simulink model "simAIDC"  (R2023b)
settings: Solver=VariableStepAuto  StartTime=0.0  StopTime=100.0  RelTol=1e-3
undefined symbols (not defined in the file or in its folder): beta, D_d, dragcoeff, G_d, gamma, K_D, K_P, Lambda, M_d, pos_init, pp, quat_init, snake, theta_init, x_init
libraries: dspindex x2
settings Model: Creator=sarava  LastModifiedBy=asker
settings SolverCC: AlgebraicLoopSolver=TrustRegion
settings DataIOCC: ReturnWorkspaceOutputs=off
settings DebuggingCC: UnconnectedInputMsg=warning  UnconnectedOutputMsg=warning  UnconnectedLineMsg=warning  ArithmeticOperatorsInVariantConditions=warning
settings ModelReferenceCC: EnableRefExpFcnMdlSchedulingChecks=on
settings SFSimCC: SimUseLocalCustomCode=off  CustomCodeUndefinedFunction=UseInterfaceOnly
settings RTWCC: RTWUseLocalCustomCode=off

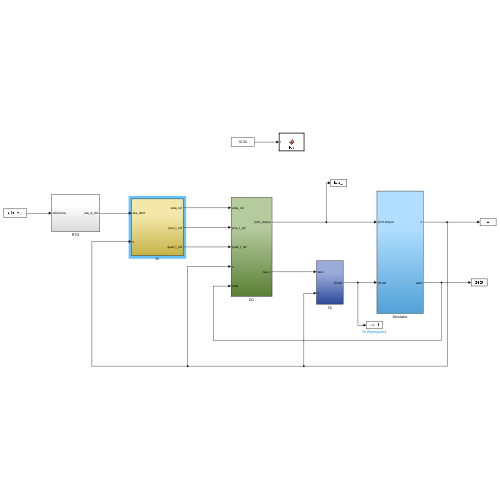
[thumbnail: Simulink's stored preview of the top-level diagram]
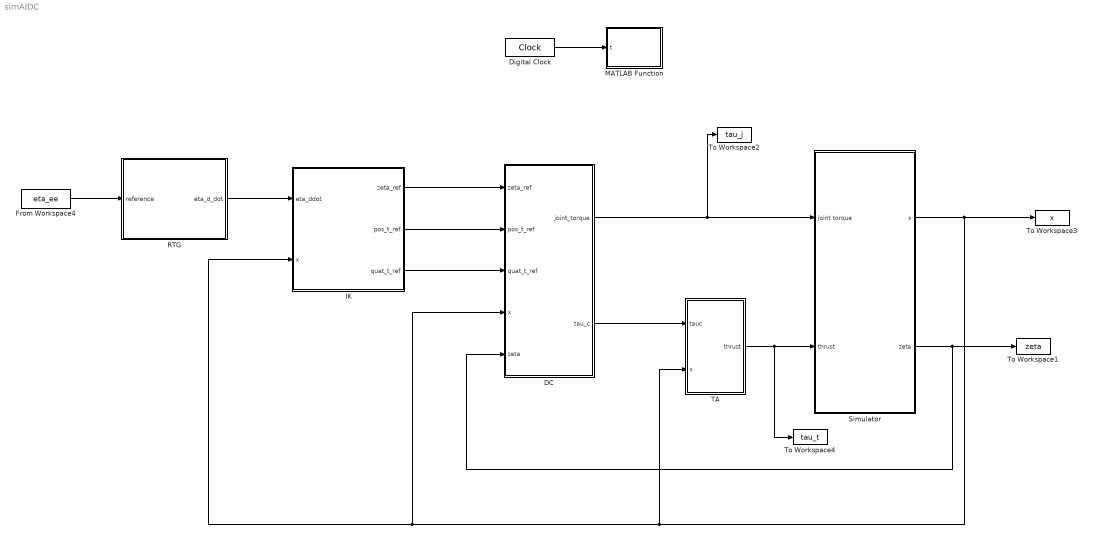
== system simAIDC ==
  DC : Subsystem
  Digital Clock : DigitalClock
  From Workspace4 : FromWorkspace  VariableName=eta_ee
  IK : Subsystem
  MATLAB Function : MATLAB Function  TreatAsAtomicUnit=on
  RTG : Subsystem
  Simulator : Subsystem
  TA : Subsystem
  To Workspace1 : ToWorkspace  VariableName=zeta  SaveFormat=Timeseries  SampleTime=-1
  To Workspace2 : ToWorkspace  VariableName=tau_j  SaveFormat=Timeseries  SampleTime=-1
  To Workspace3 : ToWorkspace  VariableName=x  SaveFormat=Timeseries  SampleTime=-1
  To Workspace4 : ToWorkspace  VariableName=tau_t  SaveFormat=Timeseries  SampleTime=-1
  wires:
  DC/2(tau_c) -> TA/1("tauc ")
  Digital Clock/1 -> MATLAB Function/1(t)
  Simulator/2(zeta) -> DC/5("zeta "), To Workspace1/1
  Simulator/1(x) -> IK/2(x), DC/4(x), TA/2("x "), To Workspace3/1
  IK/2(pos_t_ref) -> DC/2(pos_t_ref)
  IK/1(zeta_ref) -> DC/1(zeta_ref)
  IK/3(quat_t_ref) -> DC/3(quat_t_ref)
  From Workspace4/1 -> RTG/1(reference)
  RTG/1(eta_d_dot) -> IK/1(eta_ddot)
  DC/1(joint_torque) -> To Workspace2/1, Simulator/1(joint torque)
  TA/1(thrust) -> Simulator/2(thrust), To Workspace4/1

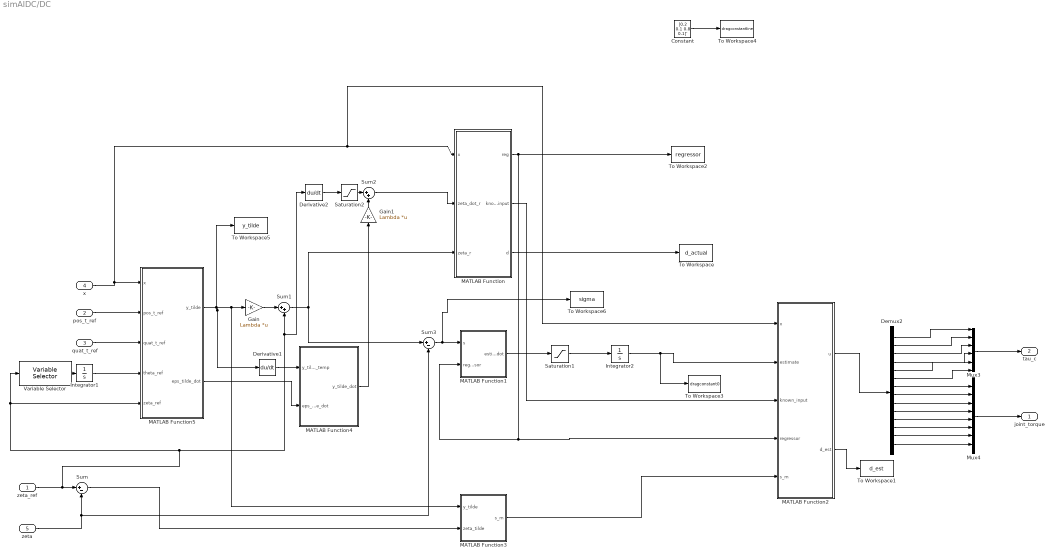
== system simAIDC/DC ==
  zeta_ref : Inport
  pos_t_ref : Inport  Port=2
  quat_t_ref : Inport  Port=3
  x : Inport  Port=4
  "zeta " : Inport  Port=5
  Constant : Constant  Value=[0.2 0.1 0.8 0.1]'
  Demux2 : Demux  Outputs=14
  Derivative1 : Derivative  CoefficientInTFapproximation=10
  Derivative2 : Derivative  CoefficientInTFapproximation=10
  Gain : Gain  Gain=Lambda  Multiplication=Matrix(K*u) (u vector)
  Gain1 : Gain  Gain=Lambda  Multiplication=Matrix(K*u) (u vector)
  Integrator1 : Integrator  InitialCondition=theta_init
  Integrator2 : Integrator  InitialCondition=[0 0 0 0]'
  MATLAB Function : MATLAB Function  TreatAsAtomicUnit=on
  MATLAB Function1 : MATLAB Function  TreatAsAtomicUnit=on
  MATLAB Function2 : MATLAB Function  TreatAsAtomicUnit=on
  MATLAB Function3 : MATLAB Function  TreatAsAtomicUnit=on
  MATLAB Function4 : MATLAB Function  TreatAsAtomicUnit=on
  MATLAB Function5 : MATLAB Function  TreatAsAtomicUnit=on
  Mux3 : Mux  Inputs=6
  Mux4 : Mux  Inputs=8
  Saturation1 : Saturate  UpperLimit=50  LowerLimit=-50  ZeroCross=off
  Saturation2 : Saturate  UpperLimit=20  LowerLimit=-20  ZeroCross=off
  Sum : Sum  Inputs=|+-
  Sum1 : Sum  Inputs=|++
  Sum2 : Sum  Inputs=|++
  Sum3 : Sum  Inputs=|+-
  To Workspace : ToWorkspace  VariableName=d_actual  SaveFormat=Timeseries  SampleTime=-1
  To Workspace1 : ToWorkspace  VariableName=d_est  SaveFormat=Timeseries  SampleTime=-1
  To Workspace2 : ToWorkspace  VariableName=regressor  SaveFormat=Timeseries  SampleTime=-1
  To Workspace3 : ToWorkspace  VariableName=dragconstant0  SaveFormat=Timeseries  SampleTime=-1
  To Workspace4 : ToWorkspace  VariableName=dragconstantline  SaveFormat=Timeseries  SampleTime=-1
  To Workspace5 : ToWorkspace  VariableName=y_tilde  SaveFormat=Timeseries  SampleTime=-1
  To Workspace6 : ToWorkspace  VariableName=sigma  SaveFormat=Timeseries  SampleTime=-1
  Variable Selector : dspindex/Variable Selector  NumInputs=1  rowsOrCols=Rows  IdxMode=Fixed  Elements=7:14  ZerOneIdxMode=One-based  errmode=Clip Index  FillMode=on  FillValues=0
  joint_torque : Outport  VectorParamsAs1DForOutWhenUnconnected=off
  tau_c : Outport  Port=2  VectorParamsAs1DForOutWhenUnconnected=off
  wires:
  x/1 -> MATLAB Function/1(x), MATLAB Function2/1(x), MATLAB Function5/1(x)
  pos_t_ref/1 -> MATLAB Function5/2(pos_t_ref)
  quat_t_ref/1 -> MATLAB Function5/3(quat_t_ref)
  zeta_ref/1 -> Derivative2/1, Sum1/2, Variable Selector/1, MATLAB Function5/5(zeta_ref), Sum/1
  "zeta "/1 -> Sum3/2, Sum/2
  Integrator1/1 -> MATLAB Function5/4(theta_ref)
  MATLAB Function5/1(y_tilde) -> MATLAB Function3/1(y_tilde), Gain/1, Derivative1/1, To Workspace5/1
  Gain/1 -> Sum1/1
  Sum1/1 -> Sum3/1, MATLAB Function/3(zeta_r)
  Saturation1/1 -> Integrator2/1
  MATLAB Function1/1(estimate_dot) -> Saturation1/1
  MATLAB Function3/1(s_m) -> MATLAB Function2/5(s_m)
  MATLAB Function2/1(u) -> Demux2/1
  Demux2/14 -> Mux4/8
  Demux2/4 -> Mux3/4
  Demux2/5 -> Mux3/5
  Demux2/12 -> Mux4/6
  Demux2/2 -> Mux3/2
  Demux2/9 -> Mux4/3
  Demux2/3 -> Mux3/3
  Demux2/13 -> Mux4/7
  Demux2/8 -> Mux4/2
  Demux2/6 -> Mux3/6
  Demux2/10 -> Mux4/4
  Demux2/7 -> Mux4/1
  Demux2/11 -> Mux4/5
  Demux2/1 -> Mux3/1
  Mux4/1 -> joint_torque/1
  Mux3/1 -> tau_c/1
  Variable Selector/1 -> Integrator1/1
  Integrator2/1 -> To Workspace3/1, MATLAB Function2/2(estimate)
  MATLAB Function/2(known_input) -> MATLAB Function2/3(known_input)
  MATLAB Function/1(reg) -> MATLAB Function1/2(regressor), MATLAB Function2/4(regressor), To Workspace2/1
  MATLAB Function5/2(eps_tilde_dot) -> MATLAB Function4/2(eps_tilde_dot)
  Derivative1/1 -> MATLAB Function4/1(y_tilde_dot_temp)
  MATLAB Function4/1(y_tilde_dot) -> Gain1/1
  Derivative2/1 -> Saturation2/1
  Saturation2/1 -> Sum2/1
  Gain1/1 -> Sum2/2
  Sum3/1 -> To Workspace6/1, MATLAB Function1/1(s)
  Sum2/1 -> MATLAB Function/2(zeta_dot_r)
  Sum/1 -> MATLAB Function3/2(zeta_tilde)
  MATLAB Function/3(d) -> To Workspace/1
  MATLAB Function2/2(d_est) -> To Workspace1/1
  Constant/1 -> To Workspace4/1

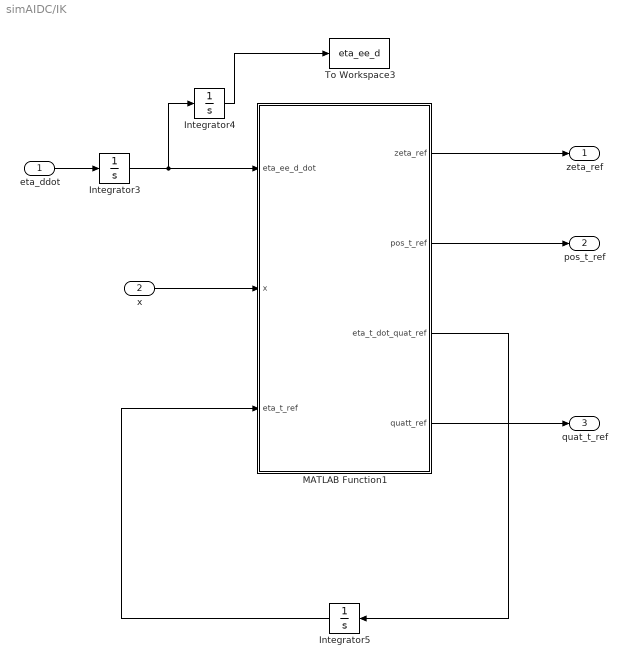
== system simAIDC/IK ==
  eta_ddot : Inport
  x : Inport  Port=2
  Integrator3 : Integrator
  Integrator4 : Integrator
  Integrator5 : Integrator  InitialCondition=[pos_init quat_init]'
  MATLAB Function1 : MATLAB Function  TreatAsAtomicUnit=on
  To Workspace3 : ToWorkspace  VariableName=eta_ee_d  SaveFormat=Timeseries  SampleTime=-1
  zeta_ref : Outport  VectorParamsAs1DForOutWhenUnconnected=off
  pos_t_ref : Outport  Port=2  VectorParamsAs1DForOutWhenUnconnected=off
  quat_t_ref : Outport  Port=3  VectorParamsAs1DForOutWhenUnconnected=off
  wires:
  MATLAB Function1/1(zeta_ref) -> zeta_ref/1
  x/1 -> MATLAB Function1/2(x)
  MATLAB Function1/2(pos_t_ref) -> pos_t_ref/1
  MATLAB Function1/3(eta_t_dot_quat_ref) -> Integrator5/1
  Integrator4/1 -> To Workspace3/1
  Integrator5/1 -> MATLAB Function1/3(eta_t_ref)
  MATLAB Function1/4(quatt_ref) -> quat_t_ref/1
  eta_ddot/1 -> Integrator3/1
  Integrator3/1 -> Integrator4/1, MATLAB Function1/1(eta_ee_d_dot)

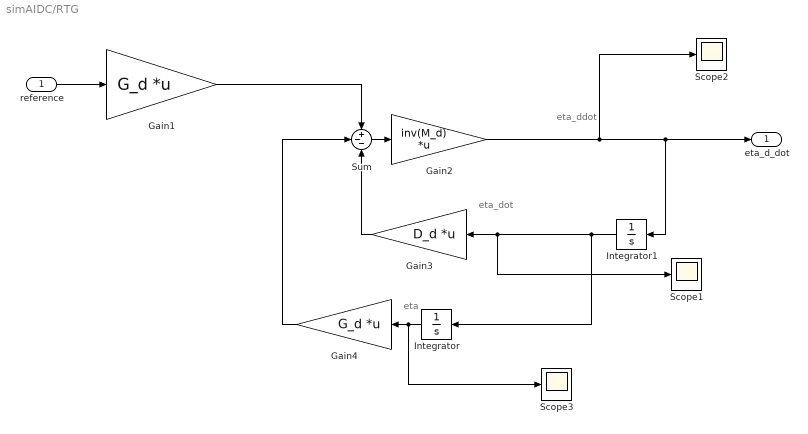
== system simAIDC/RTG ==
  note: eta_dot
  note: eta
  note: eta_ddot
  reference : Inport
  Gain1 : Gain  Gain=G_d  Multiplication=Matrix(K*u) (u vector)
  Gain2 : Gain  Gain=inv(M_d)  Multiplication=Matrix(K*u) (u vector)
  Gain3 : Gain  Gain=D_d  Multiplication=Matrix(K*u) (u vector)
  Gain4 : Gain  Gain=G_d  Multiplication=Matrix(K*u) (u vector)
  Integrator : Integrator
  Integrator1 : Integrator
  Scope1 : Scope
  Scope2 : Scope
  Scope3 : Scope
  Sum : Sum  Inputs=+--
  eta_d_dot : Outport  VectorParamsAs1DForOutWhenUnconnected=off
  wires:
  Gain2/1 -> Scope2/1, eta_d_dot/1, Integrator1/1
  Gain1/1 -> Sum/1
  Sum/1 -> Gain2/1
  reference/1 -> Gain1/1
  Integrator1/1 -> Integrator/1, Scope1/1, Gain3/1
  Integrator/1 -> Scope3/1, Gain4/1
  Gain3/1 -> Sum/3
  Gain4/1 -> Sum/2

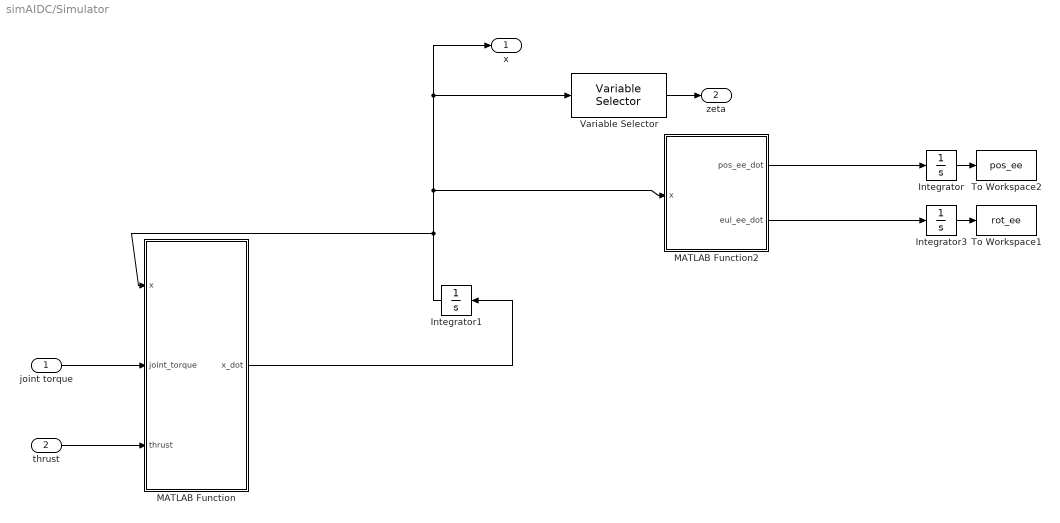
== system simAIDC/Simulator ==
  joint torque : Inport
  thrust : Inport  Port=2
  Integrator : Integrator
  Integrator1 : Integrator  InitialCondition=x_init
  Integrator3 : Integrator
  MATLAB Function : MATLAB Function  TreatAsAtomicUnit=on
  MATLAB Function2 : MATLAB Function  TreatAsAtomicUnit=on
  To Workspace1 : ToWorkspace  VariableName=rot_ee  SaveFormat=Timeseries  SampleTime=-1
  To Workspace2 : ToWorkspace  VariableName=pos_ee  SaveFormat=Timeseries  SampleTime=-1
  Variable Selector : dspindex/Variable Selector  NumInputs=1  rowsOrCols=Rows  IdxMode=Fixed  Elements=16:29  ZerOneIdxMode=One-based  errmode=Clip Index  FillMode=on  FillValues=0
  x : Outport  VectorParamsAs1DForOutWhenUnconnected=off
  zeta : Outport  Port=2  VectorParamsAs1DForOutWhenUnconnected=off
  wires:
  joint torque/1 -> MATLAB Function/2(joint_torque)
  thrust/1 -> MATLAB Function/3(thrust)
  Variable Selector/1 -> zeta/1
  MATLAB Function/1(x_dot) -> Integrator1/1
  Integrator1/1 -> Variable Selector/1, x/1, MATLAB Function2/1(x), MATLAB Function/1(x)
  Integrator/1 -> To Workspace2/1
  MATLAB Function2/1(pos_ee_dot) -> Integrator/1
  MATLAB Function2/2(eul_ee_dot) -> Integrator3/1
  Integrator3/1 -> To Workspace1/1

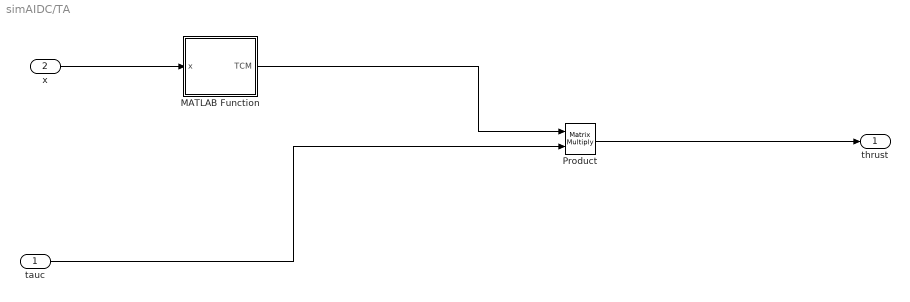
== system simAIDC/TA ==
  "tauc " : Inport
  "x " : Inport  Port=2
  MATLAB Function : MATLAB Function  TreatAsAtomicUnit=on
  Product : Product  Multiplication=Matrix(*)
  thrust : Outport  VectorParamsAs1DForOutWhenUnconnected=off
  wires:
  "x "/1 -> MATLAB Function/1(x)
  MATLAB Function/1(TCM) -> Product/1
  "tauc "/1 -> Product/2
  Product/1 -> thrust/1

== matlab function simAIDC/DC/MATLAB Function ==
  data: x input; zeta_dot_r input; reg output; known_input output; snake parameter; pp parameter; gamma parameter; beta parameter; zeta_r input; d output
function [reg, known_input,d] = regressor(x,zeta_dot_r,snake,pp, gamma, beta, zeta_r)

quat      =  x(4:7);
theta     =  x(8 : 6+snake.n);
zeta      =  x(7+snake.n : 11+2*snake.n);
[R, J]    =  comp_rot_jac(quat,theta,snake);
[c,d,g,D] = comp_cdg_adaptiv(J,R,theta,snake,pp,beta,gamma,zeta,zeta_r);
M = comp_mass(J,snake);




drag_matrix=zeros(14,4);
for i=1:snake.n
 drag_matrix=drag_matrix+J(:,:,i)'*D(:,:,i);
end



known_input= M*zeta_dot_r+c+g;

reg=drag_matrix;


end

== matlab function simAIDC/DC/MATLAB Function1 ==
  data: s input; regressor input; estimate_dot output; K_theta parameter
function estimate_dot = calc_estdot(s,regressor,K_theta)


estimate_dot=inv(K_theta)*regressor'*s;

end

== matlab function simAIDC/DC/MATLAB Function2 ==
  data: x input; estimate input; known_input input; regressor input; u output; s_m input; K_D parameter; snake parameter; d_est output
function [u,d_est]= input(x,estimate,known_input,regressor,s_m, K_D,snake)

quat      =  x(4:7);
theta     =  x(8 : 6+snake.n);

[~, J]    =  comp_rot_jac(quat,theta,snake);


B=comp_TCM(J,snake);
B_u=[eye(6,6) zeros(6,8); B(7:end,:)*pinv(B(1:6,:)) eye(8)];
d_est=regressor*estimate;
u=pinv(B_u)*(K_D*s_m+known_input+regressor*estimate);
end

== matlab function simAIDC/DC/MATLAB Function3 ==
  data: y_tilde input; zeta_tilde input; s_m output; Lambda parameter; K_D parameter; K_P parameter
function s_m = calc_estdot(y_tilde, zeta_tilde, Lambda, K_D, K_P)


s_m=zeta_tilde+Lambda*y_tilde + inv(K_D)*K_P*y_tilde;
end

== matlab function simAIDC/DC/MATLAB Function5 ==
  data: x input; y_tilde output; pos_t_ref input size=3; quat_t_ref input size=4; theta_ref input; eps_tilde_dot output; zeta_ref input
function [y_tilde,eps_tilde_dot] = dyn(x,pos_t_ref, quat_t_ref, theta_ref, zeta_ref)
pos_t=x(1:3);
quat      =  x(4:7);
theta     =  x(8 : 15);
zeta     =  x( 16: 29);

theta_tilde=theta_ref-theta;

pos_tilde=quat2rotm(quat')*(pos_t_ref-pos_t);
pos_tilde2=RotQ(quat)*(pos_t_ref-pos_t);



quat_tilde=quat(1)*quat_t_ref(2:4)-quat_t_ref(1)*quat(2:4)+cross(quat_t_ref(2:4),quat(2:4));
eta_tilde = quat(1) * quat_t_ref (1) + quat_t_ref(2:4)'*quat(2:4);

if eta_tilde < 0
quat_tilde = - quat_tilde ;
end


y_tilde=[pos_tilde;quat_tilde; theta_tilde];   %%输出1

out=pos_t_ref-pos_t;
nu2_tilde=zeta_ref(4:6)-zeta(4:6);
eps_tilde_dot=0.5*eta_tilde*nu2_tilde + 0.5*skew(quat_tilde)*nu2_tilde;  % 输出2

end

== matlab function simAIDC/Simulator/MATLAB Function ==
  data: x input; x_dot output; joint_torque input; thrust input; pp parameter; snake parameter; dragcoeff parameter
function x_dot  = dyn(x,joint_torque,thrust , pp, snake, dragcoeff)

pos       =  x(1:3);
quat      =  x(4:7);
theta     =  x(8 : 6+snake.n);
zeta      =  x(7+snake.n : 11+2*snake.n);
%Compute rotation matrices and jacobians
[Rcdg,Jcdg]=comp_rot_jac_mcdg(quat,theta,snake);
%Compute mass matrix
M         =  comp_mass(Jcdg,snake);

%Compute relative velocity to take into account the effect of current
velc_h    =  Rcdg(:,:,1)'*pp.velc;
nu        =  zeta(1:6);
zeta(1:3) =  zeta(1:3)-velc_h;

%Compute coriolis, drag, and hydrostatic terms with the relative velocity
[c, d, g] =  comp_cdg(Jcdg,Rcdg,theta,snake,pp,dragcoeff,zeta);
%Compute the thrust-configuration matrix
B         =  comp_TCM(Jcdg,snake);


%Compute the relative acceleration
zeta_dot      =  M\([B [zeros(6,8); eye(8)]]*[thrust;joint_torque]-c-d-g);% -c-d-g

%Remove the effect of current
zeta_dot(1:3) = zeta_dot(1:3)-cross(nu(4:6),velc_h);
%Compute the time derivatives of position and orientation
pos_dot   =  Rcdg(:,:,1)*nu(1:3);  
quat_dot  =  TransAngQ(quat)*nu(4:6)+1*(1-quat'*quat)*quat; 
%Assemble derivative of the state vector
x_dot = [pos_dot ; quat_dot ; zeta(7:snake.n+5) ; zeta_dot];
end

== matlab function simAIDC/MATLAB Function ==
  data: t input
function fcn(t)
%#codegen
coder.extrinsic('fprintf');
persistent firstTime

if isempty(firstTime)
    firstTime = false;
    fprintf('Starting Now\n');
end

fprintf('time = %.4f\n',t);

== matlab function simAIDC/TA/MATLAB Function ==
  data: TCM output; x input; snake parameter
function TCM = fcn(x , snake)
quat      =  x(4:7);
theta     =  x(8 : 6+snake.n);
[~, J]    =  comp_rot_jac(quat,theta,snake);
B        =  comp_TCM(J,snake);
TCM_t=B(1:6,:);
TCM=transpose(TCM_t)/(TCM_t*transpose(TCM_t));

== matlab function simAIDC/Simulator/MATLAB Function2 ==
  data: pos_ee_dot output; x input; snake parameter; eul_ee_dot output
function [pos_ee_dot, eul_ee_dot] = snake2points(x,snake)
   quat         = x(4:7);
   theta        = x(8 : 6+snake.n);
    zeta      =  x(7+snake.n : 11+2*snake.n);

   [R,J]=comp_rot_jac(quat,theta,snake);
  
   eul_ee=rotm2eul(R(:,:,10), 'XYZ')';
   Jinv=Jinv_fromeul(eul_ee);
   eta_ee_dot=[R(:,:,10) zeros(3); zeros(3) Jinv]*J(:,:,10)*zeta;
   x_ee_dot=[R(:,:,10) zeros(3); zeros(3) R(:,:,10)]*J(:,:,10)*zeta;
   pos_ee_dot=x_ee_dot(1:3);
   omega_ee=x_ee_dot(4:6);
   eul_ee_dot=eta_ee_dot(4:6);
end

== matlab function simAIDC/DC/MATLAB Function4 ==
  data: y_tilde_dot_temp input; eps_tilde_dot input; y_tilde_dot output
function y_tilde_dot = calc_estdot(y_tilde_dot_temp,eps_tilde_dot)

y_tilde_dot=[y_tilde_dot_temp(1:3);eps_tilde_dot;y_tilde_dot_temp(7:14)];
end

== matlab function simAIDC/IK/MATLAB Function1 ==
  data: eta_ee_d_dot input; x input; eta_t_ref input; zeta_ref output; snake parameter; pos_t_ref output; eta_t_dot_quat_ref output; quatt_ref output
function [zeta_ref , pos_t_ref,eta_t_dot_quat_ref, quatt_ref] = fucn(eta_ee_d_dot,x,eta_t_ref, snake)
quat      =  x(4:7);
theta     =  x(8 : 6+snake.n);
[R, J_t]    =  comp_rot_jac(quat,theta,snake);


eul_ee=rotm2eul(R(:,:,10), 'XYZ')';

Jinv=Jinv_fromeul(eul_ee);
J=[R(:,:,10) zeros(3); zeros(3) Jinv]*J_t(:,:,10);

zeta_ref=J'/(J*J'+0.0001*eye(6))*(eta_ee_d_dot);%+K*sigma_tilde);(3.3)
eta_ee_ref_dot=J*zeta_ref;%(3.2)



quatt_ref=eta_t_ref(4:7);
pos_t_ref=eta_t_ref(1:3);
R_tail=quat2rotm(quatt_ref');

pos_t_dot   =  R_tail(:,:,1)*zeta_ref(1:3);  
quat_t_dot  =  TransAngQ(quatt_ref)*zeta_ref(4:6)+1*(1-quatt_ref'*quatt_ref)*quatt_ref; 

eta_t_dot_quat_ref=[pos_t_dot; quat_t_dot];
end
